simulink model "AFM_SS_linearFDBK_obs_IMPLEMENT_outer_integral"  (R2015a)
settings: Solver=VariableStepDiscrete  StartTime=0.0  StopTime=trun  FixedStep=Ts
undefined symbols (not defined in the file): absorbDelay, C_delay, H, K, Ki, L, Nbar, Nd_out, NoiseP, Ns, PLANT, sys_obs, Ts, umax, x0_int, X0_obs
libraries: simulink x1, powerlib_meascontrol x1, customLibFcns x1, cstblocks x1
settings Model: CovSFcnEnable=off  Creator=arnold  LastModifiedBy=arnold
settings DataIOCC: LimitDataPoints=off  SaveFormat=Structure  SaveOutput=off  SaveState=on  InspectSignalLogs=on  TimeSaveName=tout_ptos
settings DebuggingCC: SolverPrmCheckMsg=warning

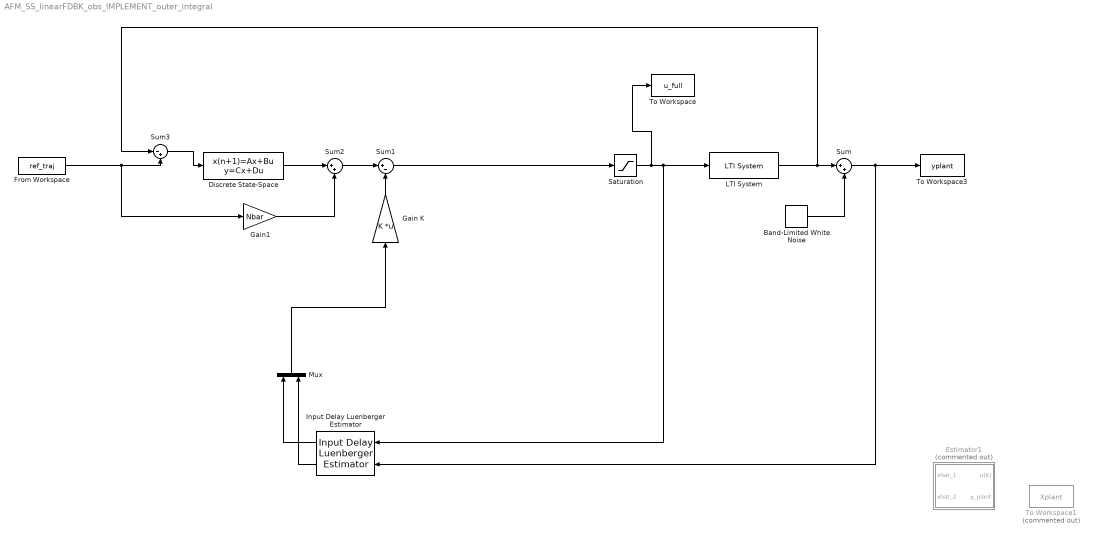
== system AFM_SS_linearFDBK_obs_IMPLEMENT_outer_integral ==
  Band-Limited White Noise : simulink/Sources/Band-Limited White Noise  Cov=[NoiseP]  Ts=Ts  seed=[23341]
  Discrete State-Space : DiscreteStateSpace  B=Ki  D=0  X0=x0_int  SampleTime=Ts
  Estimator1 : Subsystem  Commented=on
  From Workspace : FromWorkspace  VariableName=ref_traj  SampleTime=Ts
  Gain K : Gain  Gain=K  Multiplication=Matrix(K*u)
  Gain1 : Gain  Gain=Nbar
  Input Delay Luenberger Estimator : customLibFcns/Input Delay Luenberger Estimator
  LTI System : cstblocks/LTI System  sys=absorbDelay(PLANT)  IC=x0_full
  Mux : Mux  Inputs=2
  Saturation : Saturate  UpperLimit=umax  LowerLimit=-umax
  Sum : Sum  Inputs=|++
  Sum1 : Sum  Inputs=|+-
  Sum2 : Sum  Inputs=|++
  Sum3 : Sum  Inputs=|-+
  To Workspace : ToWorkspace  VariableName=u_full  SaveFormat=Timeseries  SampleTime=-1
      settings: Save2DSignal=2-D array (concatenate along first dimension)
  To Workspace1 : ToWorkspace  Commented=on  VariableName=Xplant  SaveFormat=Timeseries  SampleTime=-1
      settings: Save2DSignal=2-D array (concatenate along first dimension)
  To Workspace3 : ToWorkspace  VariableName=yplant  SaveFormat=Timeseries  SampleTime=-1
      settings: Save2DSignal=2-D array (concatenate along first dimension)
  wires:
  LTI System/1 -> Sum/1, Sum3/1
  Gain K/1 -> Sum1/2
  Input Delay Luenberger Estimator/1 -> Mux/1
  Mux/1 -> Gain K/1
  Input Delay Luenberger Estimator/2 -> Mux/2
  From Workspace/1 -> Gain1/1, Sum3/2
  Sum3/1 -> Discrete State-Space/1
  Gain1/1 -> Sum2/2
  Sum/1 -> Input Delay Luenberger Estimator/2, To Workspace3/1
  Band-Limited White Noise/1 -> Sum/2
  Saturation/1 -> To Workspace/1, Input Delay Luenberger Estimator/1, LTI System/1
  Sum1/1 -> Saturation/1
  Discrete State-Space/1 -> Sum2/1
  Sum2/1 -> Sum1/1

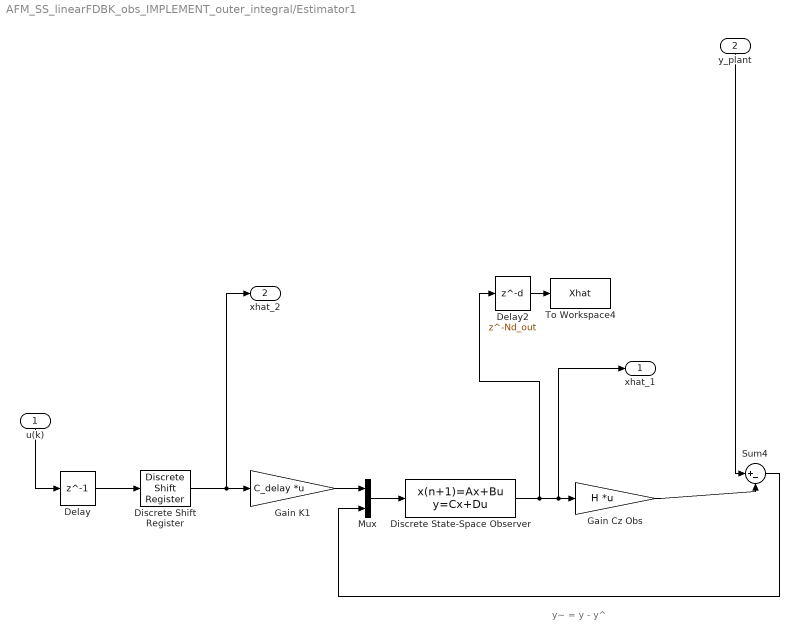
== system AFM_SS_linearFDBK_obs_IMPLEMENT_outer_integral/Estimator1 ==
  note: y~ = y - y^
  u(k) : Inport
  y_plant : Inport  Port=2
  Delay : Delay  DelayLength=1
  Delay2 : Delay  DelayLength=Nd_out
  Discrete Shift Register : powerlib_meascontrol/Additional Components/Discrete Shift Register  NSamples=Nd  InitialValue=0  Ts=Ts
  Discrete State-Space Observer : DiscreteStateSpace  A=sys_obs.a  B=[sys_obs.b, L]  C=eye(Ns)  D=zeros(Ns,2)  X0=X0_obs  SampleTime=Ts
  Gain Cz Obs : Gain  Gain=H  Multiplication=Matrix(K*u)
  Gain K1 : Gain  Gain=C_delay  Multiplication=Matrix(K*u)
  Mux : Mux  Inputs=2
  Sum4 : Sum  Inputs=|+-
  To Workspace4 : ToWorkspace  VariableName=Xhat  SaveFormat=Timeseries  SampleTime=-1
      settings: Save2DSignal=2-D array (concatenate along first dimension)
  xhat_1 : Outport
  xhat_2 : Outport  Port=2
  wires:
  Mux/1 -> Discrete State-Space Observer/1
  Sum4/1 -> Mux/2
  Discrete State-Space Observer/1 -> Delay2/1, Gain Cz Obs/1, xhat_1/1
  y_plant/1 -> Sum4/1
  Gain Cz Obs/1 -> Sum4/2
  Delay2/1 -> To Workspace4/1
  Discrete Shift Register/1 -> xhat_2/1, Gain K1/1
  Delay/1 -> Discrete Shift Register/1
  Gain K1/1 -> Mux/1
  u(k)/1 -> Delay/1
